simulink model "urban_ev_bbw_warning_logic_stateflow_validation"  (R2024b)
settings: Solver=FixedStepDiscrete  StartTime=0.0  StopTime=1  FixedStep=0.1  RelTol=1e-3
settings Model: Creator=USER  LastModifiedBy=USER

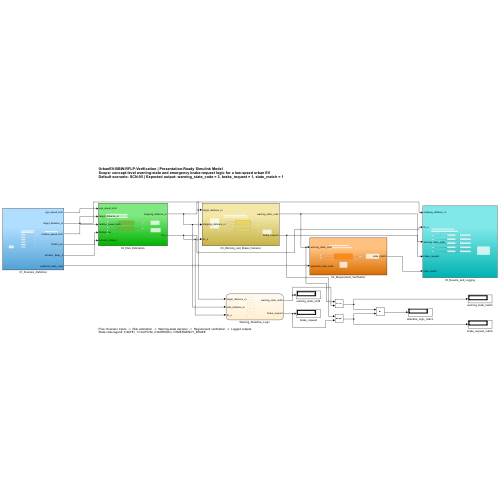
[thumbnail: Simulink's stored preview of the top-level diagram]
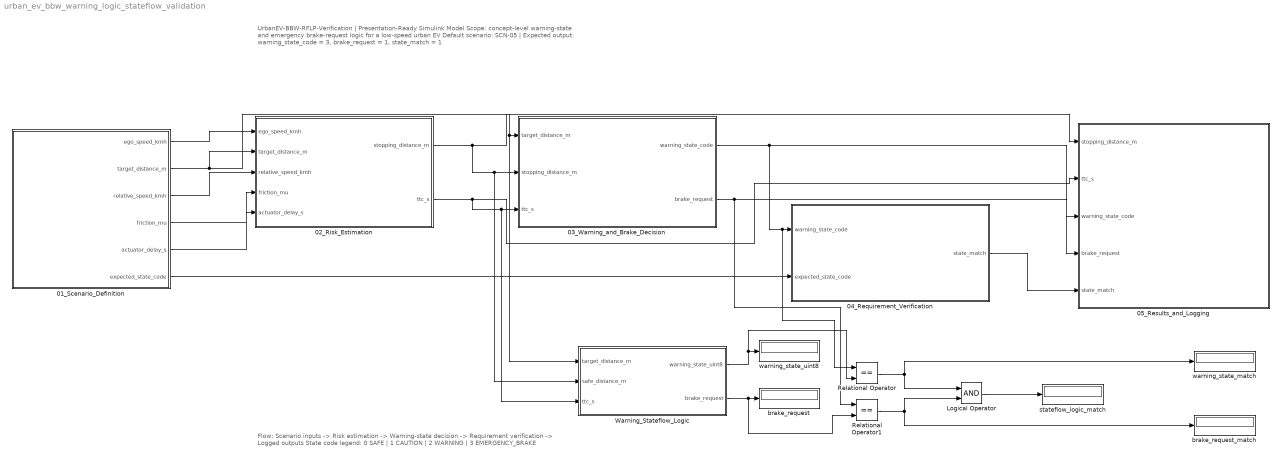
== system urban_ev_bbw_warning_logic_stateflow_validation ==
  note: UrbanEV-BBW-RFLP-Verification | Presentation-Ready Simulink Model
      | Scope: concept-level warning-state and emergency brake-request logic for a low-speed urban EV
      | Default scenario: SCN-05 | Expected output: warning_state_code = 3, brake_request = 1, state_match = 1
  note: Flow: Scenario inputs  ->  Risk estimation  ->  Warning-state decision  ->  Requirement verification  ->  Logged outputs
      | State code legend: 0 SAFE | 1 CAUTION | 2 WARNING | 3 EMERGENCY_BRAKE
  01_Scenario_Definition : Subsystem
  02_Risk_Estimation : Subsystem
  03_Warning_and_Brake_Decision : Subsystem
  04_Requirement_Verification : Subsystem
  05_Results_and_Logging : Subsystem
  Logical Operator : Logic  AllPortsSameDT=off  OutDataTypeStr=boolean
  Relational Operator : RelationalOperator  Operator===  OutDataTypeStr=boolean  RndMeth=Simplest  InputSameDT=off
  Relational Operator1 : RelationalOperator  Operator===  OutDataTypeStr=boolean  RndMeth=Simplest  InputSameDT=off
  Warning_Stateflow_Logic : Stateflow chart  TreatAsAtomicUnit=on
  brake_request : Display
  brake_request_match : Display
  stateflow_logic_match : Display
  warning_state_match : Display
  warning_state_uint8 : Display
  wires:
  01_Scenario_Definition/1(ego_speed_kmh) -> 02_Risk_Estimation/1(ego_speed_kmh)
  01_Scenario_Definition/2(target_distance_m) -> 02_Risk_Estimation/2(target_distance_m), Warning_Stateflow_Logic/1(target_distance_m), 03_Warning_and_Brake_Decision/1(target_distance_m)
  01_Scenario_Definition/3(relative_speed_kmh) -> 02_Risk_Estimation/3(relative_speed_kmh)
  01_Scenario_Definition/4(friction_mu) -> 02_Risk_Estimation/4(friction_mu)
  01_Scenario_Definition/5(actuator_delay_s) -> 02_Risk_Estimation/5(actuator_delay_s)
  02_Risk_Estimation/1(stopping_distance_m) -> Warning_Stateflow_Logic/2(safe_distance_m), 03_Warning_and_Brake_Decision/2(stopping_distance_m), 05_Results_and_Logging/1(stopping_distance_m)
  02_Risk_Estimation/2(ttc_s) -> Warning_Stateflow_Logic/3(ttc_s), 03_Warning_and_Brake_Decision/3(ttc_s), 05_Results_and_Logging/2(ttc_s)
  03_Warning_and_Brake_Decision/1(warning_state_code) -> 05_Results_and_Logging/3(warning_state_code), Relational Operator/1, 04_Requirement_Verification/1(warning_state_code)
  01_Scenario_Definition/6(expected_state_code) -> 04_Requirement_Verification/2(expected_state_code)
  03_Warning_and_Brake_Decision/2(brake_request) -> 05_Results_and_Logging/4(brake_request), Relational Operator1/1
  04_Requirement_Verification/1(state_match) -> 05_Results_and_Logging/5(state_match)
  Warning_Stateflow_Logic/1(warning_state_uint8) -> Relational Operator/2, warning_state_uint8/1
  Warning_Stateflow_Logic/2(brake_request) -> Relational Operator1/2, brake_request/1
  Relational Operator/1 -> Logical Operator/1, warning_state_match/1
  Relational Operator1/1 -> Logical Operator/2, brake_request_match/1
  Logical Operator/1 -> stateflow_logic_match/1

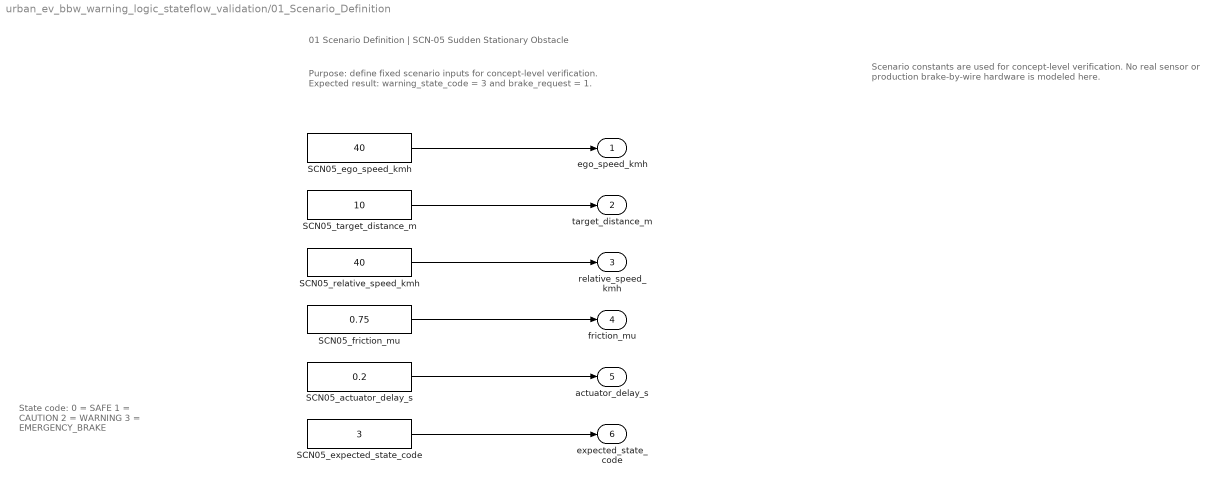
== system urban_ev_bbw_warning_logic_stateflow_validation/01_Scenario_Definition ==
  note: Scenario constants are used for concept-level verification.
      | No real sensor or production brake-by-wire hardware is modeled here.
  note: State code:
      | 0 = SAFE
      | 1 = CAUTION
      | 2 = WARNING
      | 3 = EMERGENCY_BRAKE
  note: 01 Scenario Definition | SCN-05 Sudden Stationary Obstacle
  note: Purpose: define fixed scenario inputs for concept-level verification.
      | Expected result: warning_state_code = 3 and brake_request = 1.
  SCN05_actuator_delay_s : Constant  Value=0.2
  SCN05_ego_speed_kmh : Constant  Value=40
  SCN05_expected_state_code : Constant  Value=3
  SCN05_friction_mu : Constant  Value=0.75
  SCN05_relative_speed_kmh : Constant  Value=40
  SCN05_target_distance_m : Constant  Value=10
  ego_speed_kmh : Outport
  target_distance_m : Outport  Port=2
  relative_speed_kmh : Outport  Port=3
  friction_mu : Outport  Port=4
  actuator_delay_s : Outport  Port=5
  expected_state_code : Outport  Port=6
  wires:
  SCN05_ego_speed_kmh/1 -> ego_speed_kmh/1
  SCN05_target_distance_m/1 -> target_distance_m/1
  SCN05_relative_speed_kmh/1 -> relative_speed_kmh/1
  SCN05_friction_mu/1 -> friction_mu/1
  SCN05_actuator_delay_s/1 -> actuator_delay_s/1
  SCN05_expected_state_code/1 -> expected_state_code/1

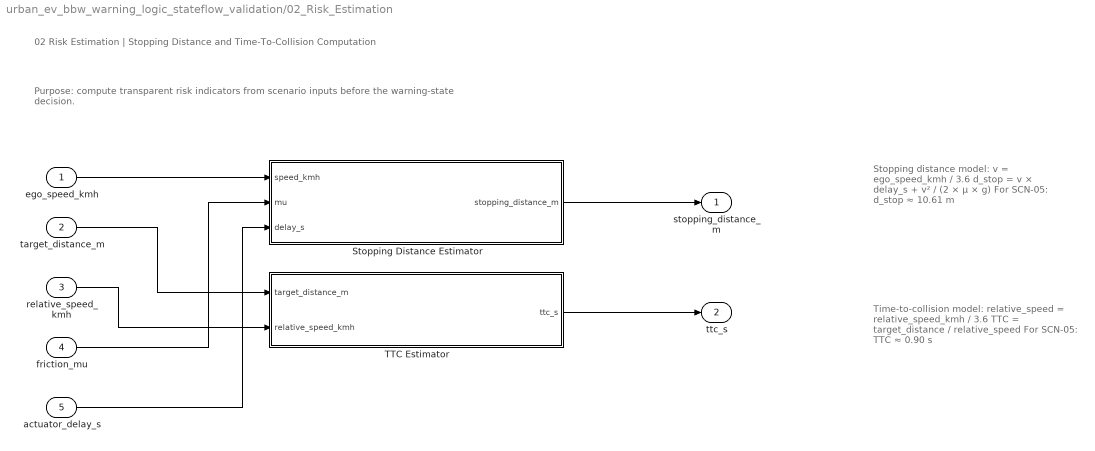
== system urban_ev_bbw_warning_logic_stateflow_validation/02_Risk_Estimation ==
  note: Time-to-collision model:
      | relative_speed = relative_speed_kmh / 3.6
      | TTC = target_distance / relative_speed
      |
      | For SCN-05:
      | TTC ≈ 0.90 s
  note: Stopping distance model:
      | v = ego_speed_kmh / 3.6
      | d_stop = v × delay_s + v² / (2 × μ × g)
      |
      | For SCN-05:
      | d_stop ≈ 10.61 m
  note: Purpose: compute transparent risk indicators from scenario inputs before the warning-state decision.
  note: 02 Risk Estimation | Stopping Distance and Time-To-Collision Computation
  ego_speed_kmh : Inport
  target_distance_m : Inport  Port=2
  relative_speed_kmh : Inport  Port=3
  friction_mu : Inport  Port=4
  actuator_delay_s : Inport  Port=5
  Stopping Distance Estimator : MATLAB Function  TreatAsAtomicUnit=on
  TTC Estimator : MATLAB Function  TreatAsAtomicUnit=on
  stopping_distance_m : Outport
  ttc_s : Outport  Port=2
  wires:
  ego_speed_kmh/1 -> Stopping Distance Estimator/1(speed_kmh)
  friction_mu/1 -> Stopping Distance Estimator/2(mu)
  actuator_delay_s/1 -> Stopping Distance Estimator/3(delay_s)
  target_distance_m/1 -> TTC Estimator/1(target_distance_m)
  relative_speed_kmh/1 -> TTC Estimator/2(relative_speed_kmh)
  Stopping Distance Estimator/1(stopping_distance_m) -> stopping_distance_m/1
  TTC Estimator/1(ttc_s) -> ttc_s/1

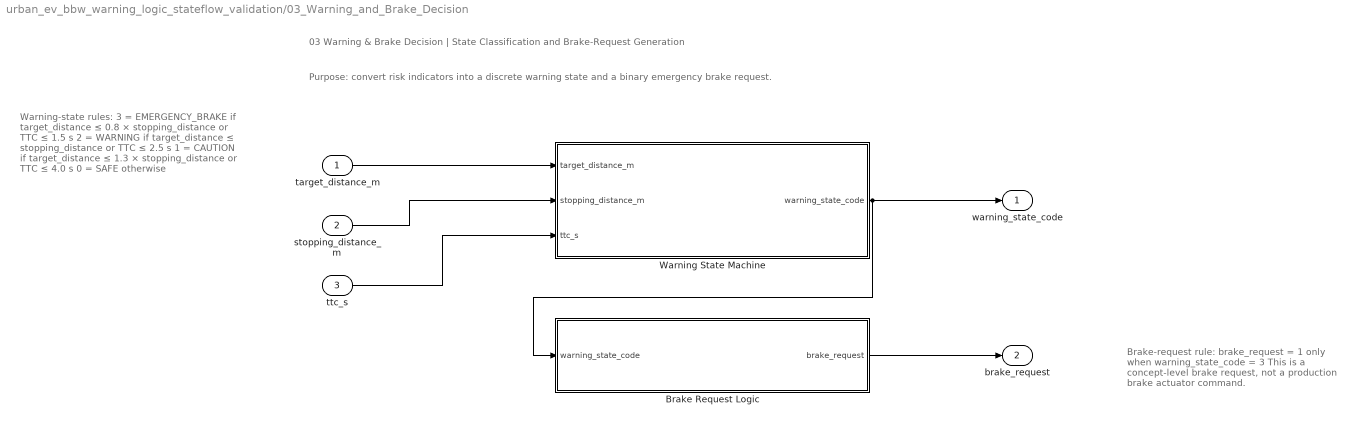
== system urban_ev_bbw_warning_logic_stateflow_validation/03_Warning_and_Brake_Decision ==
  note: Brake-request rule:
      |
      | brake_request = 1 only when
      | warning_state_code = 3
      |
      | This is a concept-level brake request,
      | not a production brake actuator command.
  note: Warning-state rules:
      |
      | 3 = EMERGENCY_BRAKE
      | if target_distance ≤ 0.8 × stopping_distance
      | or TTC ≤ 1.5 s
      |
      | 2 = WARNING
      | if target_distance ≤ stopping_distance
      | or TTC ≤ 2.5 s
      |
      | 1 = CAUTION
      | if target_distance ≤ 1.3 × stopping_distance
      | or TTC ≤ 4.0 s
      |
      | 0 = SAFE
      | otherwise
  note: 03 Warning & Brake Decision | State Classification and Brake-Request Generation
  note: Purpose: convert risk indicators into a discrete warning state and a binary emergency brake request.
  target_distance_m : Inport
  stopping_distance_m : Inport  Port=2
  ttc_s : Inport  Port=3
  Brake Request Logic : MATLAB Function  TreatAsAtomicUnit=on
  "Warning State Machine " : MATLAB Function  TreatAsAtomicUnit=on
  warning_state_code : Outport
  brake_request : Outport  Port=2
  wires:
  target_distance_m/1 -> "Warning State Machine "/1(target_distance_m)
  stopping_distance_m/1 -> "Warning State Machine "/2(stopping_distance_m)
  ttc_s/1 -> "Warning State Machine "/3(ttc_s)
  "Warning State Machine "/1(warning_state_code) -> warning_state_code/1, Brake Request Logic/1(warning_state_code)
  Brake Request Logic/1(brake_request) -> brake_request/1

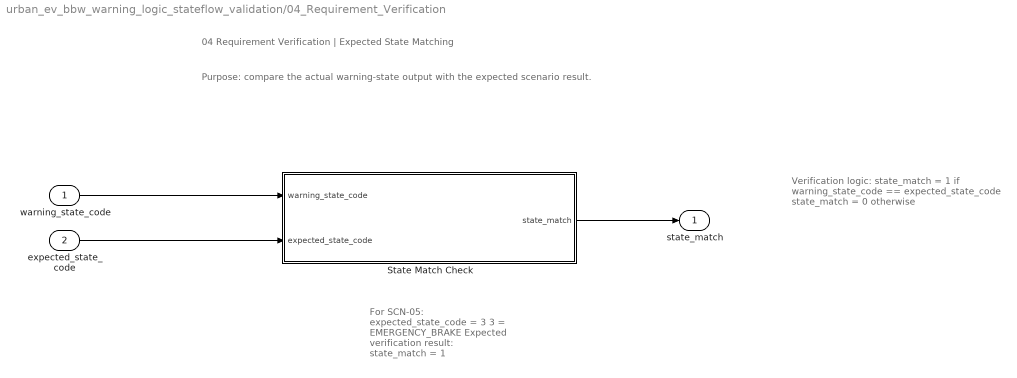
== system urban_ev_bbw_warning_logic_stateflow_validation/04_Requirement_Verification ==
  note: For SCN-05:
      | expected_state_code = 3
      |
      | 3 = EMERGENCY_BRAKE
      |
      | Expected verification result:
      | state_match = 1
  note: Verification logic:
      | state_match = 1
      | if warning_state_code == expected_state_code
      |
      | state_match = 0
      | otherwise
  note: 04 Requirement Verification | Expected State Matching
  note: Purpose: compare the actual warning-state output with the expected scenario result.
  warning_state_code : Inport
  expected_state_code : Inport  Port=2
  State Match Check : MATLAB Function  TreatAsAtomicUnit=on
  state_match : Outport
  wires:
  warning_state_code/1 -> State Match Check/1(warning_state_code)
  expected_state_code/1 -> State Match Check/2(expected_state_code)
  State Match Check/1(state_match) -> state_match/1

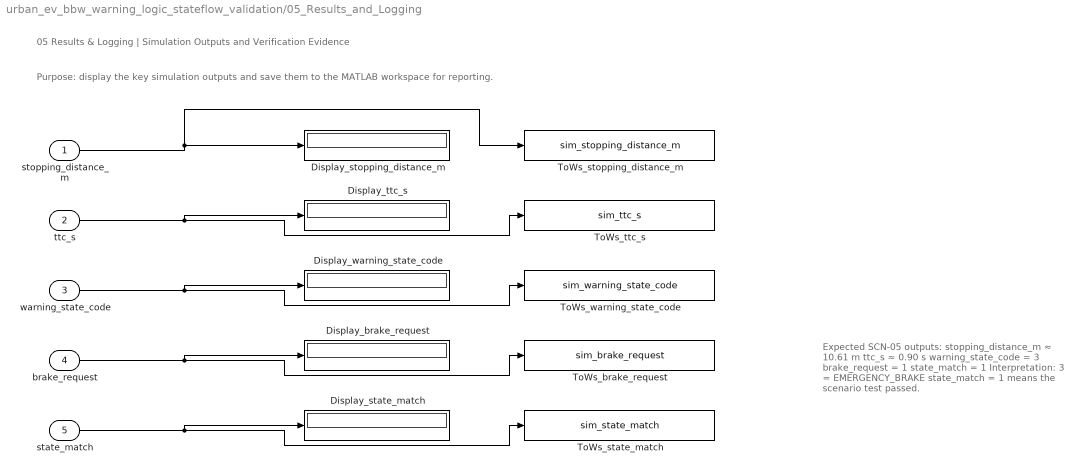
== system urban_ev_bbw_warning_logic_stateflow_validation/05_Results_and_Logging ==
  note: Expected SCN-05 outputs:
      |
      | stopping_distance_m ≈ 10.61 m
      | ttc_s ≈ 0.90 s
      | warning_state_code = 3
      | brake_request = 1
      | state_match = 1
      |
      | Interpretation:
      | 3 = EMERGENCY_BRAKE
      | state_match = 1 means the scenario test passed.
  note: 05 Results & Logging | Simulation Outputs and Verification Evidence
  note: Purpose: display the key simulation outputs and save them to the MATLAB workspace for reporting.
  stopping_distance_m : Inport
  ttc_s : Inport  Port=2
  warning_state_code : Inport  Port=3
  brake_request : Inport  Port=4
  state_match : Inport  Port=5
  Display_brake_request : Display
  Display_state_match : Display
  Display_stopping_distance_m : Display
  Display_ttc_s : Display
  Display_warning_state_code : Display
  ToWs_brake_request : ToWorkspace  VariableName=sim_brake_request  SampleTime=-1
  ToWs_state_match : ToWorkspace  VariableName=sim_state_match  SampleTime=-1
  ToWs_stopping_distance_m : ToWorkspace  VariableName=sim_stopping_distance_m  SampleTime=-1
  ToWs_ttc_s : ToWorkspace  VariableName=sim_ttc_s  SampleTime=-1
  ToWs_warning_state_code : ToWorkspace  VariableName=sim_warning_state_code  SampleTime=-1
  wires:
  stopping_distance_m/1 -> Display_stopping_distance_m/1, ToWs_stopping_distance_m/1
  ttc_s/1 -> Display_ttc_s/1, ToWs_ttc_s/1
  warning_state_code/1 -> Display_warning_state_code/1, ToWs_warning_state_code/1
  brake_request/1 -> Display_brake_request/1, ToWs_brake_request/1
  state_match/1 -> Display_state_match/1, ToWs_state_match/1

== matlab function urban_ev_bbw_warning_logic_stateflow_validation/02_Risk_Estimation/TTC Estimator ==
  data: target_distance_m input; ttc_s output; relative_speed_kmh input
function ttc_s = fcn(target_distance_m, relative_speed_kmh)
% Concept-level time-to-collision model.
relative_speed_mps = relative_speed_kmh / 3.6;
if relative_speed_mps <= 0
    ttc_s = Inf;
else
    ttc_s = target_distance_m / relative_speed_mps;
end
end

== matlab function urban_ev_bbw_warning_logic_stateflow_validation/02_Risk_Estimation/Stopping Distance Estimator ==
  data: speed_kmh input; stopping_distance_m output; mu input; delay_s input
function stopping_distance_m = fcn(speed_kmh, mu, delay_s)
% Concept-level stopping distance model
% Inputs:
% speed_kmh : ego vehicle speed [km/h]
% mu        : road friction coefficient [-]
% delay_s   : actuator/control delay [s]
%
% Equation:
% d_stop = v * delay_s + v^2 / (2 * mu * g)

g = 9.81;
v_mps = speed_kmh / 3.6;

if mu <= 0
    stopping_distance_m = Inf;
    return;
end

delay_distance_m = v_mps * delay_s;
braking_distance_m = (v_mps^2) / (2 * mu * g);

stopping_distance_m = delay_distance_m + braking_distance_m;
end

== matlab function urban_ev_bbw_warning_logic_stateflow_validation/03_Warning_and_Brake_Decision/Warning State Machine  ==
  data: target_distance_m input; warning_state_code output; stopping_distance_m input; ttc_s input
function warning_state_code = fcn(target_distance_m, stopping_distance_m, ttc_s)
% Concept-level warning-state classification
%
% State coding:
% 0 = SAFE
% 1 = CAUTION
% 2 = WARNING
% 3 = EMERGENCY_BRAKE

emergency_distance_factor = 0.8;
caution_distance_factor   = 1.3;

emergency_ttc_s = 1.5;
warning_ttc_s   = 2.5;
caution_ttc_s   = 4.0;

if target_distance_m <= emergency_distance_factor * stopping_distance_m || ttc_s <= emergency_ttc_s
    warning_state_code = 3;

elseif target_distance_m <= stopping_distance_m || ttc_s <= warning_ttc_s
    warning_state_code = 2;

elseif target_distance_m <= caution_distance_factor * stopping_distance_m || ttc_s <= caution_ttc_s
    warning_state_code = 1;

else
    warning_state_code = 0;
end
end

== matlab function urban_ev_bbw_warning_logic_stateflow_validation/03_Warning_and_Brake_Decision/Brake Request Logic ==
  data: warning_state_code input; brake_request output
function brake_request = fcn(warning_state_code)
% Concept-level emergency brake-request generation
%
% brake_request = 1 only in EMERGENCY_BRAKE state.
% This is a logical request signal, not a production actuator command.

EMERGENCY_BRAKE = 3;

brake_request = double(warning_state_code == EMERGENCY_BRAKE);
end

== matlab function urban_ev_bbw_warning_logic_stateflow_validation/04_Requirement_Verification/State Match Check ==
  data: warning_state_code input; state_match output; expected_state_code input
function state_match = fcn(warning_state_code, expected_state_code)
% Requirement verification for scenario-based testing
%
% state_match = 1 means the actual warning state matches
% the expected scenario state.
%
% State coding:
% 0 = SAFE
% 1 = CAUTION
% 2 = WARNING
% 3 = EMERGENCY_BRAKE

state_match = double(warning_state_code == expected_state_code);
end

== stateflow chart urban_ev_bbw_warning_logic_stateflow_validation/Warning_Stateflow_Logic ==
  state SAFE
    du:
    warning_state_uint8 = uint8(0);
    brake_request = false;
  state CAUTION
    du:
    warning_state_uint8 = uint8(1);
    brake_request = false;
  state WARNING
    du:
    warning_state_uint8 = uint8(2);
    brake_request = false;
  state EMERGENCY_BRAKE
    du:
    warning_state_uint8 = uint8(3);
    brake_request = true;
  (default) -> SAFE
  SAFE -> CAUTION : [target_distance_m <= 1.3*safe_distance_m || ttc_s <= 3.5]
  CAUTION -> WARNING : [target_distance_m <= safe_distance_m || ttc_s <= 2.0]
  WARNING -> EMERGENCY_BRAKE : [ttc_s <= 1.5 || target_distance_m <= 0.7*safe_distance_m]
  data: warning_state_uint8 output uint8 size=1; brake_request output boolean size=1; target_distance_m input size=1; safe_distance_m input size=1; ttc_s input size=1
